simulink model "ZenerClipper"  (R2015a)
settings: Solver=ode23tb  StartTime=0.0  StopTime=0.05  RelTol=1e-3
libraries: powerlib x16, simulink x1
settings Model: Creator=asus  LastModifiedBy=asus

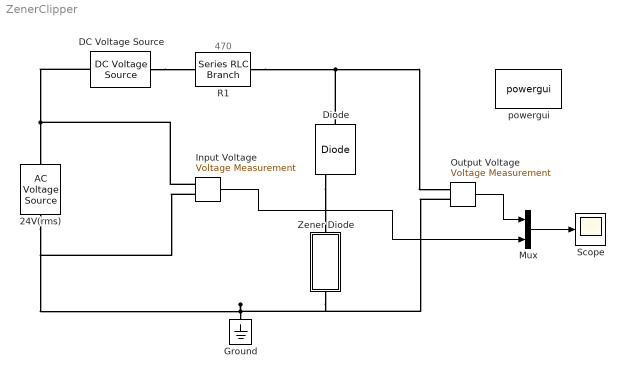
== system ZenerClipper ==
  note: 470
  24V(rms) : powerlib/Electrical Sources/AC Voltage Source  Amplitude=24*sqrt(2)  Phase=0  Frequency=60  SampleTime=0  Measurements=Voltage
  DC Voltage Source : powerlib/Electrical Sources/DC Voltage Source  Amplitude=10  Measurements=Voltage
  Diode : powerlib/Power Electronics/Diode  Ron=0.001  Lon=0  Vf=0.8  IC=0  UseSnubber=off  Rs=0  Cs=0  Measurements=on
  Ground : powerlib/Elements/Ground  LConnTagsString=a
  Input Voltage : powerlib/Measurements/Voltage Measurement  PhasorSimulation=off  OutputType=Complex  PSBequivalent=0
  Mux : Mux  Inputs=2
  Output Voltage : powerlib/Measurements/Voltage Measurement  PhasorSimulation=off  OutputType=Complex  PSBequivalent=0
  R1 : powerlib/Elements/Series RLC Branch  LConnTagsString=__new0  RConnTagsString=__new0  BranchType=R  Resistance=470  Inductance=1e-3  SetiL0=off  InitialCurrent=0  Capacitance=1e-6  Setx0=off  InitialVoltage=0  Measurements=None
  Scope : Scope
      settings: YMin=-15  YMax=15
  Zener Diode : Subsystem  mask(Zener Diode){Vz=10, Rzt=10, Rzk=400, Izm=400e-3, Vf=0.7, Ron=1e-3}
      mask prompts: Vz "Zener Voltage Vz (V)"; Rzt "Dynamic Impedance Zzt (ohms)"; Rzk "Knee Impedance Zzk (ohms)"; Izm "Maximum Continuous Current Izm (A)"; Vf "Forward Voltage Drop Vf (V)"; Ron "On Resistance Ron (ohms)"
      mask help:
      | Implements a zener diode block.
      | Use values from standard datasheets to populate block dialog
  powergui : powerlib/powergui  Priority=1  SimulationMode=Continuous  SolverType=Tustin/Backward Euler (TBE)  SampleTime=10e-6  frequency=60  SPID=on  DisableSnubberDevices=on  DisableRonSwitches=off  DisableVfSwitches=off  SwTol=0  DisplayEquations=off  Interpol=off  methode=off  Ts=100  FunctionMessages=off  echomessages=off  HookPort=off  EnableUseOfTLC=off  x0status=blocks  frequencyindice=0  Pbase=100e6  ErrMax=1e-4  Iterations=50  UnitsV=kV  UnitsW=MW  buscounter=0  RestoreLinks=warning  ResistiveCurrentMeasurement=off  Frange=[0:2:500]  Ylog=off  Xlog=on  ShowGrid=off  save=off  variable=ZData  structure=0  ZoomFFT=off  StartTime=0.0  cycles=1  DisplayStyle=1  fundamental=60  FreqAxis=off  MaxFrequency=1000  frequencyindicesteady=1  RmsSteady=1  display=off
  wires:
  Input Voltage/1 -> Mux/2
  Output Voltage/1 -> Mux/1
  Mux/1 -> Scope/1
  connections:
  Ground/LConn1 -- Input Voltage/LConn2 -- 24V(rms)/LConn1 -- Zener Diode/RConn1 -- Output Voltage/LConn2
  R1/RConn1 -- Diode/LConn1 -- Output Voltage/LConn1
  Input Voltage/LConn1 -- 24V(rms)/RConn1 -- DC Voltage Source/RConn1
  DC Voltage Source/LConn1 -- R1/LConn1
  Diode/RConn1 -- Zener Diode/LConn1

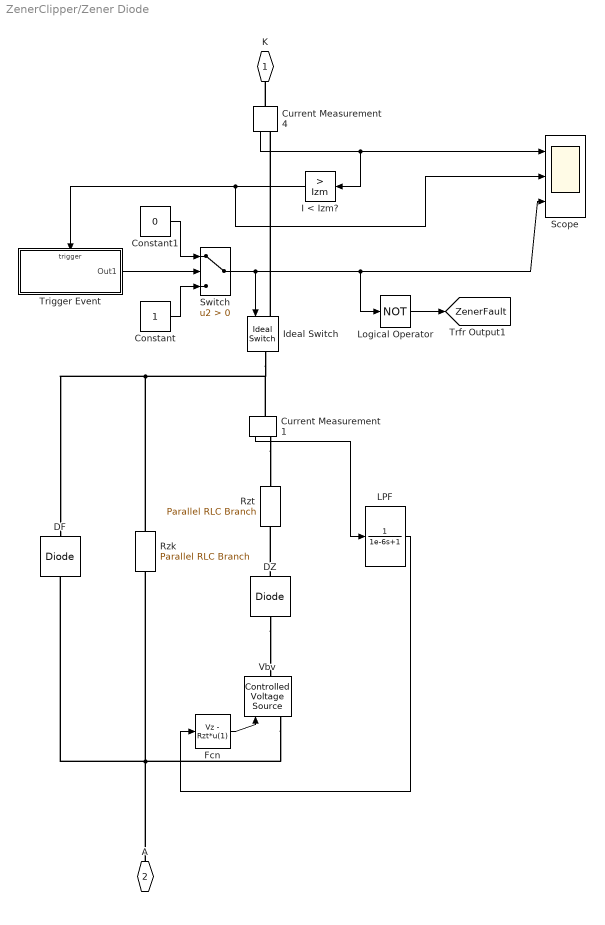
== system ZenerClipper/Zener Diode ==
  Constant : Constant
  Constant1 : Constant  Value=0
  Current Measurement1 : powerlib/Measurements/Current Measurement  PhasorSimulation=off  OutputType=Complex  PSBequivalent=0
  Current Measurement4 : powerlib/Measurements/Current Measurement  PhasorSimulation=off  OutputType=Complex  PSBequivalent=0
  DF : powerlib/Power Electronics/Diode  Ron=Ron  Lon=0  Vf=Vf  IC=0  UseSnubber=off  Rs=1000  Cs=0  Measurements=off
  DZ : powerlib/Power Electronics/Diode  Ron=1e-6  Lon=0  Vf=0  IC=0  UseSnubber=off  Rs=100  Cs=inf  Measurements=off
  Fcn : Fcn  Expr=Vz - Rzt*u(1)
  I < Izm? : simulink/Logic and Bit Operations/Compare To Constant  relop=>  const=Izm  OutDataTypeStr=boolean
  Ideal Switch : powerlib/Power Electronics/Ideal Switch  Ron=0.001  Lon=0  IC=1  Rs=1e5  Cs=0  Measurements=off
  LPF : TransferFcn  Denominator=[1e-6 1]
  Logical Operator : Logic  Operator=NOT  AllPortsSameDT=off  OutDataTypeStr=boolean
  Rzk : powerlib/Elements/Parallel RLC Branch  LConnTagsString=a  RConnTagsString=__new0  BranchType=R  Resistance=Rzk  Inductance=1.0  SetiL0=off  InitialCurrent=0  Capacitance=1e-5  Setx0=off  InitialVoltage=0  Measurements=None
  Rzt : powerlib/Elements/Parallel RLC Branch  LConnTagsString=a  RConnTagsString=__new0  BranchType=R  Resistance=Rzt  Inductance=1.0  SetiL0=off  InitialCurrent=0  Capacitance=1e-5  Setx0=off  InitialVoltage=0  Measurements=None
  Scope : Scope  NumInputPorts=3
      settings: YMin=-2.77556e-017~-1~0.95  YMax=0.4~1~1.05  SaveName=ScopeData4
  Switch : Switch  Criteria=u2 > Threshold
  Trigger Event : Subsystem  TreatAsAtomicUnit=on
  Vbv : powerlib/Electrical Sources/Controlled Voltage Source  Initialize=off  Source_Type=DC  Amplitude=0  Phase=0  Frequency=0  Measurements=None
  K : PMIOPort  Port=1  Side=Left
  A : PMIOPort  Port=2  Side=Right
  tag scope: ZenerFault=global
  wires:
  Fcn/1 -> Vbv/1
  Current Measurement4/1 -> Scope/1, I < Izm?/1
  Current Measurement1/1 -> LPF/1
  LPF/1 -> Fcn/1
  I < Izm?/1 -> Scope/2, Trigger Event/Trigger
  Switch/1 -> Ideal Switch/1, Scope/3, Logical Operator/1
  Trigger Event/1(Out1) -> Switch/2
  Constant/1 -> Switch/3
  Constant1/1 -> Switch/1
  Logical Operator/1 -> [ZenerFault]
  connections:
  DZ/RConn1 -- Vbv/RConn1
  Current Measurement4/LConn1 -- K/RConn1
  DZ/LConn1 -- Rzt/LConn1
  Current Measurement1/RConn1 -- Rzt/RConn1
  Rzk/RConn1 -- Current Measurement1/LConn1 -- Ideal Switch/RConn1 -- DF/RConn1
  Ideal Switch/LConn1 -- Current Measurement4/RConn1
  A/RConn1 -- DF/LConn1 -- Rzk/LConn1 -- Vbv/LConn1

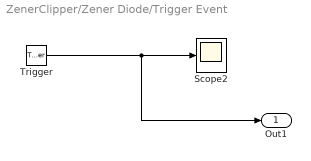
== system ZenerClipper/Zener Diode/Trigger Event ==
  Trigger : TriggerPort  ShowOutputPort=on
  Scope2 : Scope
      settings: YMin=-1  YMax=1
  Out1 : Outport
  wires:
  Trigger/1 -> Scope2/1, Out1/1
